simulink model "GalvoModel_v31_TEST_CC"  (R2013a)
settings: Solver=ode45  StartTime=0.0  StopTime=30e-3  RelTol=1e-3
undefined symbols (not defined in the file or in its folder): Kp_cc
libraries: simulink x1
settings Model: Creator=mainster  LastModifiedBy=mainster
settings DebuggingCC: SolverPrmCheckMsg=none

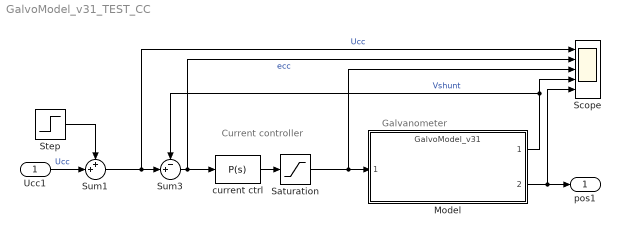
== system GalvoModel_v31_TEST_CC ==
  note: Current controller
  note: Galvanometer
  Ucc1 : Inport
  Model : ModelReference  ModelNameDialog=GalvoModel_v31.slx  SimulationMode=Normal  ModelReferenceVersion=1.9  CopyOfModelName=GalvoModel_v31.slx  DefaultDataLogging=on
      mask Display:
      | str=sprintf('%s',get(gcbh,'ModelName'));
      | port_label('input', 1, 'VCoil','texmode','on')
      | color('blue');
      | port_label('output', 1, 'VShunt','texmode','on')
      | color('black');
      | port_label('output', 2, 'AngPos')
      | %text(.05,.98,['{\fontsize{12}\it\bf' strrep(str,'_',' ') '}'],'horizontalAlignment','left','verticalAlignment','top','texmode','on')
      | text(.05,.98,['{\fontsize{12}\it\bf' strrep(str,'_','\_') '}'],'horizontalAlignment','left','verticalAlignment','top','texmode','on')
      | 
      | %get_param(gcbh,'Location')
      | % pos = get_param(gcb, 'Position');
      | % width = pos(3) - pos(1);
      | % x = [0, width];
      | % y = ones(1,length(x))*0.8;
      | % plot(x,y)
  Saturation : Saturate  UpperLimit=25  LowerLimit=-25
      settings: AttributesFormatString=Saturation:\n<%<LowerLimit>\n>%<UpperLimit>
  Scope : Scope  NumInputPorts=5
      settings: ShowLegends=on  TimeRange=0.03  YMin=0~0~0~0~0  YMax=0.1~0.1~0.05~0.004~0.006  MaxDataPoints=500000
  Step : Step  Time=1e-3  After=0.1  SampleTime=0
  Sum1 : Sum  Inputs=++|
  Sum3 : Sum  Inputs=-+|
  current ctrl : simulink/Continuous/PID Controller  Controller=P  TimeDomain=Continuous-time  SampleTime=1  IntegratorMethod=Forward Euler  FilterMethod=Forward Euler  Form=Parallel  P=Kp_cc  I=0.7525  D=0.156  N=100  InitialConditionSource=internal  InitialConditionForIntegrator=0  InitialConditionForFilter=0  ExternalReset=none  LimitOutput=off  UpperSaturationLimit=25  LowerSaturationLimit=-25  LinearizeAsGain=off  AntiWindupMode=none  Kb=1  TrackingMode=off  Kt=1  PParamMin=[]  PParamMax=[]  IParamMin=[]  IParamMax=[]  DParamMin=[]  DParamMax=[]  NParamMin=[]  NParamMax=[]  KbParamMin=[]  KbParamMax=[]  KtParamMin=[]  KtParamMax=[]  POutMin=[]  POutMax=[]  IOutMin=[]  IOutMax=[]  DOutMin=[]  DOutMax=[]  NOutMin=[]  NOutMax=[]  KbOutMin=[]  KbOutMax=[]  KtOutMin=[]  KtOutMax=[]  IntegratorOutMin=[]  IntegratorOutMax=[]  FilterOutMin=[]  FilterOutMax=[]  SumOutMin=[]  SumOutMax=[]  SumI1OutMin=[]  SumI1OutMax=[]  SumI2OutMin=[]  SumI2OutMax=[]  SumI3OutMin=[]  SumI3OutMax=[]  SumDOutMin=[]  SumDOutMax=[]  SaturationOutMin=[]  SaturationOutMax=[]  IntegratorContinuousStateAttributes=''  IntegratorStateMustResolveToSignalObject=off  IntegratorRTWStateStorageClass=Auto  FilterContinuousStateAttributes=''  FilterStateMustResolveToSignalObject=off  FilterRTWStateStorageClass=Auto
  pos1 : Outport
  wires:
  Model/2 -> Scope/5, pos1/1
  Sum3/1 -> Scope/2, current ctrl/1  "ecc"
  current ctrl/1 -> Saturation/1
  Saturation/1 -> Scope/3, Model/1
  Model/1 -> Scope/4, Sum3/1  "Vshunt"
  Ucc1/1 -> Sum1/2  "Ucc"
  Sum1/1 -> Scope/1, Sum3/2  "Ucc"
  Step/1 -> Sum1/1
